simulink library "x2RelHum"  (R2018b)
settings: Solver=ode45  StartTime=0.0  StopTime=10.0  RelTol=1e-3  EnableMultiTasking=on
libraries: carnot x1
settings Model: Creator=lena.frank  LastModifiedBy=P41573
settings DataIOCC: LimitDataPoints=on  SaveFormat=Array  SignalLoggingSaveFormat=ModelDataLogs
settings OptimizationCC: ExpressionDepthLimit=2147483647  LifeSpan=inf
settings DebuggingCC: UnderspecifiedInitializationDetection=Classic  MergeDetectMultiDrivingBlocksExec=none  SolverPrmCheckMsg=warning  FcnCallInpInsideContextMsg=warning  StateNameClashWarn=warning  SFUnexpectedBacktrackingDiag=warning  SFNoUnconditionalDefaultTransitionDiag=warning  SFExecutionAtInitializationDiag=none
settings HardwareCC: ProdBitPerPointer=32  ProdBitPerSizeT=32  ProdBitPerPtrDiffT=32  ProdLargestAtomicFloat=None  ProdIntDivRoundTo=Undefined  ProdEndianess=Unspecified  ProdWordSize=32  ProdHWDeviceType=32-bit Generic
settings ModelReferenceCC: PropagateSignalLabelsOutOfModel=off
settings SFSimCC: SimUseLocalCustomCode=off
settings RTWCC: RTWUseLocalCustomCode=off
settings CodeAppCC: StateflowObjectComments=on
settings GRTTargetCC: TargetLangStandard=C89/C90 (ANSI)  GeneratePreprocessorConditionals=Disable all  CombineOutputUpdateFcns=off  GRTInterface=on
settings ConfigComp: CovMetricSettings=dw  CovHtmlReporting=on  CovSaveCumulativeToWorkspaceVar=on  CovSaveSingleToWorkspaceVar=on  CovExternalEMLEnable=off

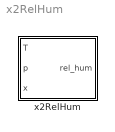
== system x2RelHum ==
  x2RelHum : Subsystem  mask(x to relative humidity){}
      mask help:
      | Calculate  the relative humidity of air
      | from the mass of water per mass of air (x).
      |
      | T             [°C]
      | p             [Pa]
      | rel_hum   [percent]
      | x              kg water / kg dry air
      mask Help: web(fullfile(path_carnot('help'),'x2rel_hum.html'),'-helpbrowser')

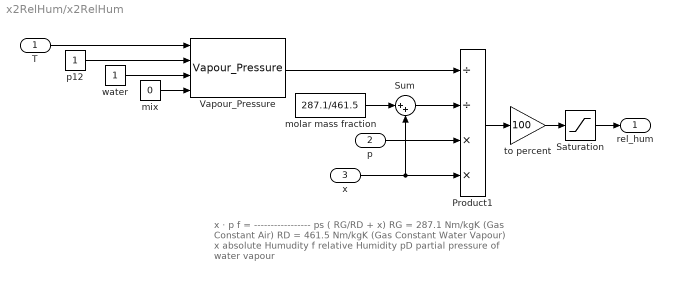
== system x2RelHum/x2RelHum ==
  note: x · p
      | f =  -----------------
      |         ps ( RG/RD + x)
      |
      | RG = 287.1 Nm/kgK (Gas Constant Air)
      | RD = 461.5 Nm/kgK (Gas Constant Water Vapour)
      | x absolute Humudity
      | f relative Humidity
      | pD partial pressure of water vapour
  T : Inport
  p : Inport  Port=2
  x : Inport  Port=3
  Product1 : Product  Inputs=//**  SaturateOnIntegerOverflow=on  InputSameDT=on  OutDataTypeStr=Inherit: Same as first input
  Saturation : Saturate  UpperLimit=100  LowerLimit=0
  Sum : Sum  Inputs=|++  SaturateOnIntegerOverflow=on  InputSameDT=on  OutDataTypeStr=Inherit: Same as first input
  Vapour_Pressure : carnot/Basic/Material_Properties/Vapour_Pressure  VariantControl=CarlibClassic  INPUTARGUMENTS=state variables (classic)  DEBUGLEVEL=WARNINGLEVEL  MAXTOTALMESSAGES=inf  MAXCONSECUTIVEMESSAGES=inf  WRITETOFILE=0  FILENAME='errors.txt'
      settings: SourceProductName=Carnot
  mix : Constant  Value=0
  "molar mass fraction " : Constant  Value=287.1/461.5
  p12 : Constant
  to percent : Gain  Gain=100  SaturateOnIntegerOverflow=on  OutDataTypeStr=Inherit: Same as input  ParamDataTypeStr=Inherit: Same as input
  water : Constant
  rel_hum : Outport
  wires:
  "molar mass fraction "/1 -> Sum/1
  Saturation/1 -> rel_hum/1
  to percent/1 -> Saturation/1
  Vapour_Pressure/1 -> Product1/1
  Sum/1 -> Product1/2
  p/1 -> Product1/3
  x/1 -> Product1/4, Sum/2
  Product1/1 -> to percent/1
  T/1 -> Vapour_Pressure/1
  water/1 -> Vapour_Pressure/3
  p12/1 -> Vapour_Pressure/2
  mix/1 -> Vapour_Pressure/4
